simulink model "control_simulation"  (R2018a)
settings: Solver=ode8  StartTime=0.0  StopTime=sm_time  FixedStep=Ts  RelTol=1e-3
values from neighbouring files (symbols this model uses):
  J = 0.0017    [main_simulation_code.m]
  Ki = 35    [main_simulation_code.m]
  Kp = 70    [main_simulation_code.m]
  kr = Lm/Lr    (= 0.966040361865)    [main_simulation_code.m]
  Lm = 0.6941    [main_simulation_code.m]
  p = 2    [main_simulation_code.m]
  r_sigma = Rs+kr^2*Rr    (= 12.0114932716)    [main_simulation_code.m]
  T_nom = 4.1    [main_simulation_code.m]
  t_sigma = sigma*Ls/r_sigma    (= 0.00399379025945)    [main_simulation_code.m]
  t_T = TorqueTable(:,1)    [main_simulation_code.m]
  t_w = SpeedTable(:,1)    [main_simulation_code.m]
  tr = Lr/Rr    (= 0.148699269439)    [main_simulation_code.m]
  Tref = TorqueTable(:,2)    [main_simulation_code.m]
  Ts = 1e-5    (= 1e-05)    [main_simulation_code.m]
  Vdc = 520    [main_simulation_code.m]
  wref = SpeedTable(:,2)    [main_simulation_code.m]
undefined symbols (not defined in the file or in its folder): DiscIntNeverNeededParam, j
libraries: powerlib_meascontrol x1
settings Model: Creator=eduar  LastModifiedBy=eduar

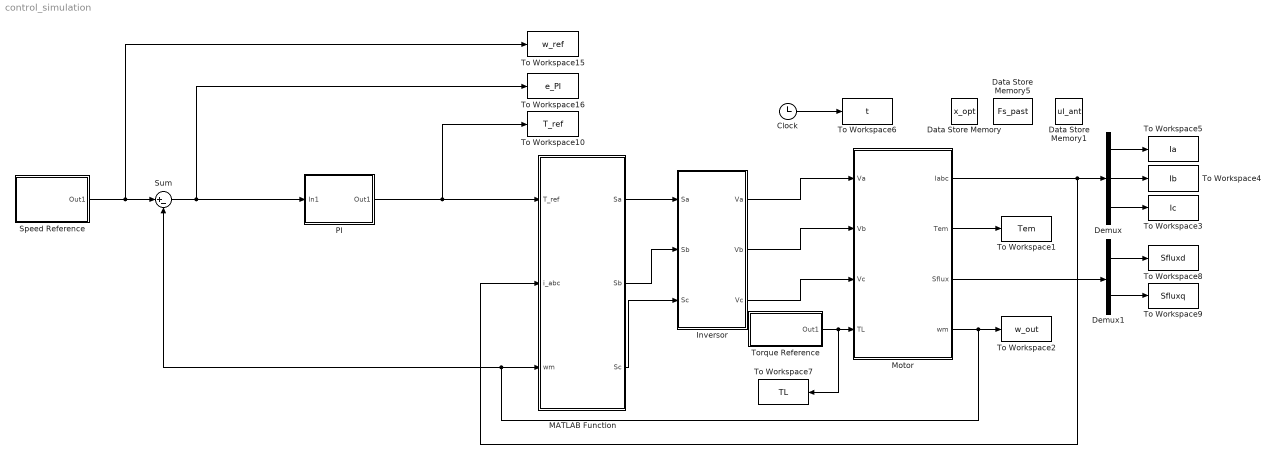
== system control_simulation ==
  Clock : Clock
  Data Store Memory : DataStoreMemory  DataStoreName=x_opt  InitialValue=1  ShowAdditionalParam=off  OutDataTypeStr=double
  Data Store Memory1 : DataStoreMemory  DataStoreName=uI_ant  InitialValue=1  ShowAdditionalParam=off  OutDataTypeStr=double
  Data Store Memory5 : DataStoreMemory  DataStoreName=Fs_past  InitialValue=0 + 0*sqrt(-1)*1;  ShowAdditionalParam=off  OutDataTypeStr=double
      settings: SignalType=complex
  Demux : Demux  Outputs=3
  Demux1 : Demux  Outputs=2
  Inversor : Subsystem
  MATLAB Function : MATLAB Function  TreatAsAtomicUnit=on
  Motor : Subsystem
  PI : Subsystem
  Speed Reference : Subsystem
  Sum : Sum  Inputs=|+-
  To Workspace1 : ToWorkspace  VariableName=Tem  SampleTime=-1
  To Workspace10 : ToWorkspace  VariableName=T_ref  SampleTime=-1
  To Workspace15 : ToWorkspace  VariableName=w_ref  SampleTime=-1
  To Workspace16 : ToWorkspace  VariableName=e_PI  SampleTime=-1
  To Workspace2 : ToWorkspace  VariableName=w_out  SampleTime=-1
  To Workspace3 : ToWorkspace  VariableName=Ic  SampleTime=-1
  To Workspace4 : ToWorkspace  VariableName=Ib  SampleTime=-1
  To Workspace5 : ToWorkspace  VariableName=Ia  SampleTime=-1
  To Workspace6 : ToWorkspace  VariableName=t  SampleTime=-1
  To Workspace7 : ToWorkspace  VariableName=TL  SampleTime=-1
  To Workspace8 : ToWorkspace  VariableName=Sfluxd  SampleTime=-1
  To Workspace9 : ToWorkspace  VariableName=Sfluxq  SampleTime=-1
  Torque Reference : Subsystem
  wires:
  MATLAB Function/1(Sa) -> Inversor/1(Sa)
  MATLAB Function/2(Sb) -> Inversor/2(Sb)
  MATLAB Function/3(Sc) -> Inversor/3(Sc)
  Clock/1 -> To Workspace6/1
  Sum/1 -> PI/1(In1), To Workspace16/1
  Inversor/1(Va) -> Motor/1(Va)
  Inversor/2(Vb) -> Motor/2(Vb)
  Inversor/3(Vc) -> Motor/3(Vc)
  Motor/4(wm) -> Sum/2, MATLAB Function/3(wm), To Workspace2/1
  Torque Reference/1(Out1) -> To Workspace7/1, Motor/4(TL)
  Motor/1(Iabc) -> MATLAB Function/2(i_abc), Demux/1
  Motor/2(Tem) -> To Workspace1/1
  Demux/3 -> To Workspace3/1
  Demux/2 -> To Workspace4/1
  Demux/1 -> To Workspace5/1
  Motor/3(Sflux) -> Demux1/1
  Demux1/2 -> To Workspace9/1
  Demux1/1 -> To Workspace8/1
  Speed Reference/1(Out1) -> Sum/1, To Workspace15/1
  PI/1(Out1) -> To Workspace10/1, MATLAB Function/1(T_ref)

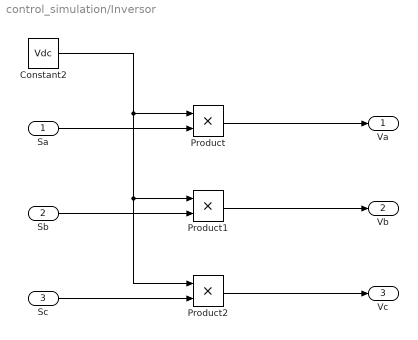
== system control_simulation/Inversor ==
  Sa : Inport
  Sb : Inport  Port=2
  Sc : Inport  Port=3
  Constant2 : Constant  Value=Vdc
  Product : Product
  Product1 : Product
  Product2 : Product
  Va : Outport
  Vb : Outport  Port=2
  Vc : Outport  Port=3
  wires:
  Sb/1 -> Product1/2
  Constant2/1 -> Product2/1, Product1/1, Product/1
  Sa/1 -> Product/2
  Product1/1 -> Vb/1
  Product2/1 -> Vc/1
  Sc/1 -> Product2/2
  Product/1 -> Va/1

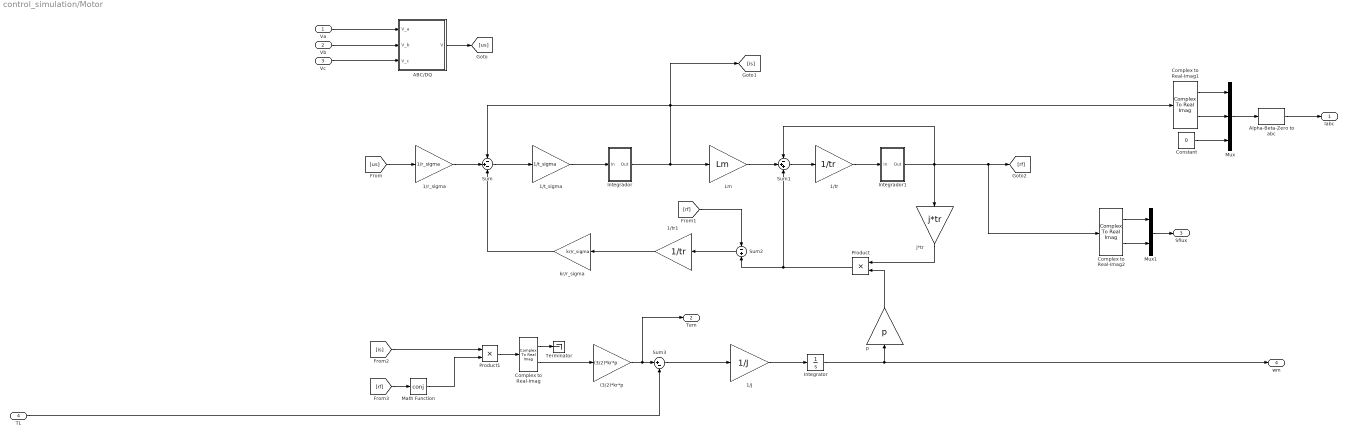
== system control_simulation/Motor ==
  Va : Inport
  Vb : Inport  Port=2
  Vc : Inport  Port=3
  TL : Inport  Port=4
  (3/2)*kr*p : Gain  Gain=(3/2)*kr*p
  1/J : Gain  Gain=1/J
  1/r_sigma : Gain  Gain=1/r_sigma
  "1/t_sigma " : Gain  Gain=1/t_sigma
  1/tr : Gain  Gain=1/tr
  1/tr1 : Gain  Gain=1/tr
  ABC/DQ : MATLAB Function  TreatAsAtomicUnit=on
  Alpha-Beta-Zero to abc : powerlib_meascontrol/Transformations/Alpha-Beta-Zero to abc
      settings: SourceProductName=Simscape Power Systems  SourceProductBaseCode=PS
  Complex to Real-Imag : ComplexToRealImag
  Complex to Real-Imag1 : ComplexToRealImag
  Complex to Real-Imag2 : ComplexToRealImag
  Constant : Constant  Value=0
  Integrador : Subsystem
  Integrador1 : Subsystem
  Integrator : Integrator
  Lm : Gain  Gain=Lm
  Math Function : Math  Operator=conj  SaturateOnIntegerOverflow=on
  Mux : Mux  Inputs=3
  Mux1 : Mux  Inputs=2
  Product : Product
  Product1 : Product
  Sum : Sum  Inputs=-+-
  Sum1 : Sum  Inputs=-++
  Sum2 : Sum  Inputs=-+
  Sum3 : Sum  Inputs=|+-
  Terminator : Terminator
  j*tr : Gain  Gain=j*tr
  kr/r_sigma : Gain  Gain=kr/r_sigma
  p : Gain  Gain=p
  Iabc : Outport
  Tem : Outport  Port=2
  Sflux : Outport  Port=3
  wm : Outport  Port=4
  wires:
  Complex to Real-Imag/2 -> (3/2)*kr*p/1
  j*tr/1 -> Product/1
  Integrator/1 -> wm/1, p/1
  Sum3/1 -> 1/J/1
  Va/1 -> ABC/DQ/1(V_a)
  p/1 -> Product/2
  1/tr/1 -> Integrador1/1(In)
  Lm/1 -> Sum1/2
  (3/2)*kr*p/1 -> Tem/1, Sum3/1
  Sum/1 -> "1/t_sigma "/1
  kr/r_sigma/1 -> Sum/3
  Sum1/1 -> 1/tr/1
  Product1/1 -> Complex to Real-Imag/1
  [rf] -> Math Function/1
  Math Function/1 -> Product1/2
  ABC/DQ/1(V) -> [us]
  "1/t_sigma "/1 -> Integrador/1(In)
  Sum2/1 -> 1/tr1/1
  Product/1 -> Sum1/3, Sum2/2
  [rf] -> Sum2/1
  [is] -> Product1/1
  1/tr1/1 -> kr/r_sigma/1
  1/J/1 -> Integrator/1
  1/r_sigma/1 -> Sum/2
  [us] -> 1/r_sigma/1
  TL/1 -> Sum3/2
  Vb/1 -> ABC/DQ/2(V_b)
  Vc/1 -> ABC/DQ/3(V_c)
  Complex to Real-Imag/1 -> Terminator/1
  Mux/1 -> Alpha-Beta-Zero to abc/1
  Integrador/1(Out) -> Lm/1, Complex to Real-Imag1/1, Sum/1, [is]
  Complex to Real-Imag1/2 -> Mux/2
  Complex to Real-Imag1/1 -> Mux/1
  Alpha-Beta-Zero to abc/1 -> Iabc/1
  Constant/1 -> Mux/3
  Complex to Real-Imag2/2 -> Mux1/2
  Complex to Real-Imag2/1 -> Mux1/1
  Mux1/1 -> Sflux/1
  Integrador1/1(Out) -> Sum1/1, j*tr/1, Complex to Real-Imag2/1, [rf]

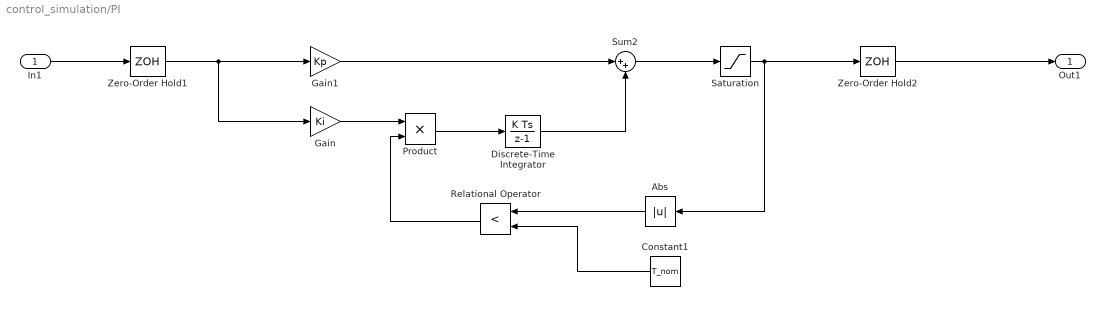
== system control_simulation/PI ==
  In1 : Inport
  Abs : Abs
  Constant1 : Constant  Value=T_nom
  Discrete-Time Integrator : DiscreteIntegrator  SampleTime=-1  ICPrevOutput=DiscIntNeverNeededParam  ICPrevScaledInput=DiscIntNeverNeededParam
  Gain : Gain  Gain=Ki
  Gain1 : Gain  Gain=Kp
  Product : Product
  Relational Operator : RelationalOperator  Operator=<  OutDataTypeStr=boolean  RndMeth=Simplest
  Saturation : Saturate  UpperLimit=T_nom  LowerLimit=-T_nom
  Sum2 : Sum  Inputs=|++
  Zero-Order Hold1 : ZeroOrderHold  SampleTime=Ts
  Zero-Order Hold2 : ZeroOrderHold  SampleTime=Ts
  Out1 : Outport
  wires:
  Sum2/1 -> Saturation/1
  Zero-Order Hold1/1 -> Gain/1, Gain1/1
  Gain/1 -> Product/1
  Saturation/1 -> Zero-Order Hold2/1, Abs/1
  Gain1/1 -> Sum2/1
  Constant1/1 -> Relational Operator/2
  Abs/1 -> Relational Operator/1
  Relational Operator/1 -> Product/2
  Discrete-Time Integrator/1 -> Sum2/2
  Product/1 -> Discrete-Time Integrator/1
  Zero-Order Hold2/1 -> Out1/1
  In1/1 -> Zero-Order Hold1/1

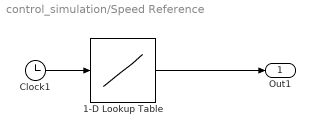
== system control_simulation/Speed Reference ==
  1-D Lookup Table : Lookup_n-D  NumberOfTableDimensions=1  BreakpointsForDimension1=t_w  Table=wref  InternalRulePriority=Speed  RndMeth=Simplest  InputSameDT=on
  Clock1 : Clock
  Out1 : Outport
  wires:
  Clock1/1 -> 1-D Lookup Table/1
  1-D Lookup Table/1 -> Out1/1

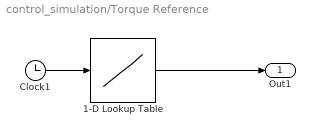
== system control_simulation/Torque Reference ==
  1-D Lookup Table : Lookup_n-D  NumberOfTableDimensions=1  BreakpointsForDimension1=t_T  Table=Tref  InterpMethod=Nearest  InternalRulePriority=Speed  RndMeth=Simplest  InputSameDT=on
  Clock1 : Clock
  Out1 : Outport
  wires:
  Clock1/1 -> 1-D Lookup Table/1
  1-D Lookup Table/1 -> Out1/1

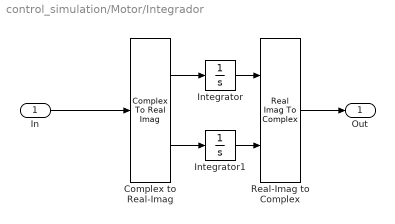
== system control_simulation/Motor/Integrador ==
  In : Inport
  Complex to Real-Imag : ComplexToRealImag
  Integrator : Integrator
  Integrator1 : Integrator
  Real-Imag to Complex : RealImagToComplex
  Out : Outport
  wires:
  Integrator/1 -> Real-Imag to Complex/1
  Real-Imag to Complex/1 -> Out/1
  Integrator1/1 -> Real-Imag to Complex/2
  Complex to Real-Imag/1 -> Integrator/1
  In/1 -> Complex to Real-Imag/1
  Complex to Real-Imag/2 -> Integrator1/1

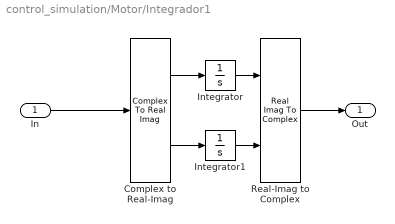
== system control_simulation/Motor/Integrador1 ==
  In : Inport
  Complex to Real-Imag : ComplexToRealImag
  Integrator : Integrator
  Integrator1 : Integrator
  Real-Imag to Complex : RealImagToComplex
  Out : Outport
  wires:
  Integrator/1 -> Real-Imag to Complex/1
  Real-Imag to Complex/1 -> Out/1
  Integrator1/1 -> Real-Imag to Complex/2
  Complex to Real-Imag/1 -> Integrator/1
  In/1 -> Complex to Real-Imag/1
  Complex to Real-Imag/2 -> Integrator1/1

== matlab function control_simulation/Motor/ABC//DQ ==
  data: V_a input; V output; V_b input; V_c input
function V  = fcn(V_a, V_b, V_c)
V = (2/3)*(V_a + exp(j*(2*pi/3))*V_b + exp(j*(4*pi/3))*V_c);

== matlab function control_simulation/MATLAB Function ==
  settings: updateMethod=DISCRETE  sampleTime=Ts
  data: T_ref input; Sa output double size=1; i_abc input; wm input; Sb output double size=1; Sc output double size=1; x_opt data_store_memory; Fs_past data_store_memory; param parameter; uI_ant data_store_memory
function [Sa, Sb, Sc] = control(T_ref, i_abc, wm, param)
    % Variables defined in the parameters file
    global x_opt Fs_past uI_ant
    Ts = param.Ts; Rs = param.Rs; Lr = param.Lr;
    Lm = param.Lm; Ls = param.Ls; p = param.p;
    tr = param.tr; kr = param.kr; r_sigma = param.r_sigma;
    t_sigma = param.t_sigma; lambda = param.lambda;
    v = param.v; states = param.states;
    sf_nom = param.sf_nom;
   
    
    V_k = v(x_opt);
    %Calcula a corrente
    i_meas = (2/3)*(i_abc(1) + exp(j*(2*pi/3))*i_abc(2) + exp(j*(4*pi/3))*i_abc(3));
    
    % Stator flux estimate
    Fs_k = Fs_past + Ts*(V_k - Rs*i_meas);
    Fs_past = Fs_k;
    % Rotor flux estimate
    Fr = (Lr/Lm)*Fs_k + i_meas*(Lm - (Lr*Ls)/Lm);
    g_opt = 1e10;
    for i = 1:8
        % i-th voltage vector for current prediction
        v_o1 = v(i);
        % Stator current prediction at instant k+1
        Isp1 = (1 + (Ts/t_sigma))*i_meas + (Ts/(t_sigma + Ts))*((1/r_sigma)*(((kr/tr) - kr*j*wm)*Fs_k + v_o1));
        
        % Stator flux prediction at instant k+1
        Fsp1 = Fs_k + Ts*v_o1 - Rs*Ts*i_meas;
        
        % Torque prediction at instant k+1
        Tp1 = (3/2)*p*imag(conj(Fsp1)*Isp1);
        
        % Cost function
        g = abs(T_ref - Tp1)+ lambda*abs(sf_nom-abs(Fsp1));
        
        if (g<g_opt)
            g_opt = g;
            x_opt = i;
        end
        
    end
    % Output switching states
    Sa = states(x_opt,1);
    Sb = states(x_opt,2);
    Sc = states(x_opt,3);
